simulink model "STEVE_ver28"  (R2022a)
settings: Solver=VariableStepAuto  StartTime=0.0  StopTime=Stop_Time  FixedStep=0.000001  RelTol=1e-5
values from neighbouring files (symbols this model uses):
  Bed_ave_OD = (1+Bed_ins_OD)/2    (= 1.667)    [STEVE_initialization.m]    (also in STEVE_running.m = (1+Bed_ins_OD)/2; STEVE_v4_C1Demo_2023_Nominal.m)
  Bed_ins_OD = 2.334    [STEVE_initialization.m]    (also in STEVE_v4_C1Demo_2023_Nominal.m)
  Bed_thickness = 0.049    [STEVE_initialization.m]    (also in STEVE_v4_C1Demo_2023_Nominal.m)
  Belimo_Cv = 16    [STEVE_initialization.m]    (also in STEVE_v4_C1Demo_2023_Nominal.m)
  flow_rate = 8    [STEVE_initialization.m]    (also in STEVE_v4_C1Demo_2023_Nominal.m)
  Heat_ads = 40000    [STEVE_initialization.m]    (also in STEVE_v4_C1Demo_2023_Nominal.m)
  Heater_output = 85.3    [STEVE_initialization.m]    (also in STEVE_v4_C1Demo_2023_Nominal.m)
  L = 0.508    [STEVE_initialization.m]    (also in STEVE_v4_C1Demo_2023_Nominal.m)
  L_inch = L*39.3701    (= 20.0000108)    [STEVE_initialization.m]    (also in STEVE_v4_C1Demo_2023_Nominal.m)
  max_temp = 200+273.15    (= 473.15)    [STEVE_initialization.m]    (also in STEVE_v4_C1Demo_2023_Nominal.m)
  mesh_size = 15    [STEVE_initialization.m]    (also in STEVE_v4_C1Demo_2023_Nominal.m)
  Pipe_ave_HD = (pipe_HD+0.5)/2    (= 0.465)    [STEVE_initialization.m]    (also in STEVE_running.m = (pipe_HD+0.5)/2; STEVE_v4_C1Demo_2023_Nominal.m)
  pipe_HD = 0.43    [STEVE_initialization.m]    (also in STEVE_v4_C1Demo_2023_Nominal.m)
  Ramp_rate = 0.0833    [STEVE_initialization.m]    (also in STEVE_v4_C1Demo_2023_Nominal.m)
  room_pressure = 13.3    [STEVE_initialization.m]    (also in STEVE_v4_C1Demo_2023_Nominal.m)
  t_Total = Adsorption_time + FlowStop_time + Valve_close_Time + Select_valve_close_Time + Pump_down_time + Desorption_time + SelectValve_open_Time + Valve_open_Time    (= 9635)    [STEVE_initialization.m]    (also in STEVE_running.m = Adsorption_time + FlowStop_time + Valve_close_Time + Select_; STEVE_v4_C1Demo_2023_Nominal.m)
libraries: fl_lib x229, nesl_utility x75, slpidlib x2
(part 3 of 5)

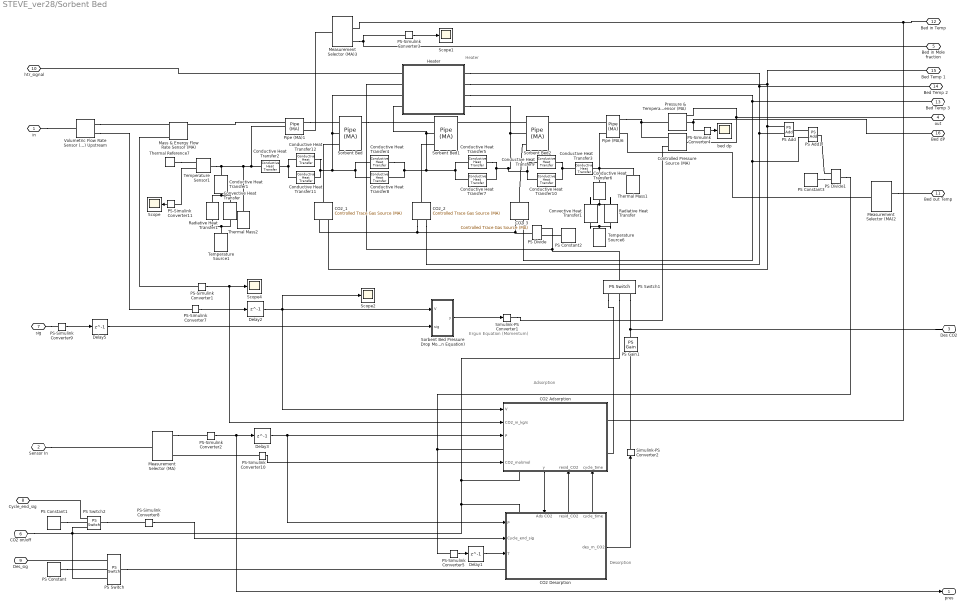
== system STEVE_ver28/Sorbent Bed ==
  note: Adsorption
  note: Desorption
  note: Heater
  note: Ergun Equation
      | (Momentum)
  CO2 Adsorption : Subsystem
      settings: PortSchema="{\"entries\":[{\"content\":{\"sides\":[{\"content\":{\"connectorIds\":[\"In1\",\"In2\",\"In3\",\"LConn1\",\"In4\"]},\"type\":\"ConnectorPlacement.EquallySpacedRectSide\",\"uuid\":\"fb5d8689-8c7c-41c6-b33a-026ebdfeda46\"},{\"content\":{\"connectorIds\":[\"RConn1\",\"RConn2\"],\"side\":\"RIGHT\"},\"type\":\"ConnectorPlacement.EquallySpacedRectSide\",\"uuid\":\"e615a398-5db1-42bf-ba80-688914a64f02\"},{\"content\":{\"connectorIds\":[],\"side\":\"TOP\"},\"type\":\"ConnectorPlacement.EquallySpacedRectSide\",\"uuid\":\"9c645526-20b8-4187-b1de-a01e982b301c\"},{\"content\":{\"connectorIds\":[\"RConn3\",\"Out1\",\"In5\",\"In6\"],\"side\":\"BOTTOM\"},\"type\":\"ConnectorPlacement.EquallySpacedRectSide\",\"uuid\":\"6466ec51-34c2-43b0-b46d-13f7eb07024c\"}]},\"type\":\"ConnectorPlacement.EquallySpacedConnector\",\"uuid\":\"b40ef80e-51c9-40d8-be75-3e6ecf2a6433\"}],\"packageUris\":[\"http://schema.mathworks.com/mf0/Connector/R2020b\"],\"version\":\"1.0\"}"
  CO2 Desorption : Subsystem
      settings: PortSchema="{\"entries\":[{\"content\":{\"sides\":[{\"content\":{\"connectorIds\":[\"In1\",\"In2\",\"In3\",\"LConn1\"]},\"type\":\"ConnectorPlacement.EquallySpacedRectSide\",\"uuid\":\"c0a19cc0-55b6-4f26-88f6-d4532b770ac9\"},{\"content\":{\"connectorIds\":[\"Out1\"],\"side\":\"RIGHT\"},\"type\":\"ConnectorPlacement.EquallySpacedRectSide\",\"uuid\":\"04c46a21-a116-4a66-b667-6b06cdc38df3\"},{\"content\":{\"connectorIds\":[\"LConn2\",\"In4\",\"Out2\",\"Out3\"],\"side\":\"TOP\"},\"type\":\"ConnectorPlacement.EquallySpacedRectSide\",\"uuid\":\"2474eb99-1ff9-473d-8974-056a2586b2d8\"}]},\"type\":\"ConnectorPlacement.EquallySpacedConnector\",\"uuid\":\"155b9182-f960-4b43-b6e5-30b3ea77ead6\"}],\"packageUris\":[\"http://schema.mathworks.com/mf0/Connector/R2020b\"],\"version\":\"1.0\"}"
  CO2_1 : fl_lib/Moist Air/Sources/Moisture & Trace Gas Sources/Controlled Trace Gas Source (MA)  Phi_S_specify=off  Phi_S_priority=None  Phi_S=0 kW  Phi_S_nominal_specify=off  Phi_S_nominal_unit=kW  Phi_S_nominal_value=1  mdot_g_S_specify=off  mdot_g_S_priority=None  mdot_g_S=0 kg/s  mdot_g_S_nominal_specify=off  mdot_g_S_nominal_unit=kg/s  mdot_g_S_nominal_value=1
      settings: SourceProductBaseCode=PW,SS,VE  InternalSimscapePortConfiguration="{\"Bottom\":[],\"Left\":[{\"id\":\"S\",\"label\":\"S\",\"type\":\"foundation.moist_air.moist_air_source\"}],\"Right\":[{\"id\":\"M\",\"label\":\"M\",\"type\":\"input\"},{\"id\":\"T\",\"label\":\"T\",\"type\":\"input\"}],\"Top\":[]}"
  CO2_2 : fl_lib/Moist Air/Sources/Moisture & Trace Gas Sources/Controlled Trace Gas Source (MA)  Phi_S_specify=off  Phi_S_priority=None  Phi_S=0 kW  Phi_S_nominal_specify=off  Phi_S_nominal_unit=kW  Phi_S_nominal_value=1  mdot_g_S_specify=off  mdot_g_S_priority=None  mdot_g_S=0 kg/s  mdot_g_S_nominal_specify=off  mdot_g_S_nominal_unit=kg/s  mdot_g_S_nominal_value=1
      settings: SourceProductBaseCode=PW,SS,VE  InternalSimscapePortConfiguration="{\"Bottom\":[],\"Left\":[{\"id\":\"S\",\"label\":\"S\",\"type\":\"foundation.moist_air.moist_air_source\"}],\"Right\":[{\"id\":\"M\",\"label\":\"M\",\"type\":\"input\"},{\"id\":\"T\",\"label\":\"T\",\"type\":\"input\"}],\"Top\":[]}"
  CO2_3 : fl_lib/Moist Air/Sources/Moisture & Trace Gas Sources/Controlled Trace Gas Source (MA)  Phi_S_specify=off  Phi_S_priority=None  Phi_S=0 kW  Phi_S_nominal_specify=off  Phi_S_nominal_unit=kW  Phi_S_nominal_value=1  mdot_g_S_specify=off  mdot_g_S_priority=None  mdot_g_S=0 kg/s  mdot_g_S_nominal_specify=off  mdot_g_S_nominal_unit=kg/s  mdot_g_S_nominal_value=1
      settings: SourceProductBaseCode=PW,SS,VE  InternalSimscapePortConfiguration="{\"Bottom\":[],\"Left\":[{\"id\":\"S\",\"label\":\"S\",\"type\":\"foundation.moist_air.moist_air_source\"}],\"Right\":[{\"id\":\"M\",\"label\":\"M\",\"type\":\"input\"},{\"id\":\"T\",\"label\":\"T\",\"type\":\"input\"}],\"Top\":[]}"
  Conductive Heat Transfer1 : fl_lib/Thermal/Thermal Elements/Conductive Heat Transfer  area=2*pi*(1.531/2)*1.2 in^2  thickness=(1.531-Bed_thickness*2-pipe_HD)/2 in  th_cond=pipe_tc W/(m*K)  T_specify=off  T_priority=None  T=0 K  T_nominal_specify=off  T_nominal_unit=K  T_nominal_value=1  Q_specify=off  Q_priority=None  Q=0 W  Q_nominal_specify=off  Q_nominal_unit=W  Q_nominal_value=1
      settings: SourceProductBaseCode=PW,SS,VE
  Conductive Heat Transfer10 : fl_lib/Thermal/Thermal Elements/Conductive Heat Transfer  area=pi*(0.902/2)^2 in^2  thickness=20/3 in  th_cond=0.15 W/(m*K)  T_specify=off  T_priority=None  T=0 K  T_nominal_specify=off  T_nominal_unit=K  T_nominal_value=1  Q_specify=off  Q_priority=None  Q=0 W  Q_nominal_specify=off  Q_nominal_unit=W  Q_nominal_value=1
      settings: SourceProductBaseCode=PW,SS,VE
  Conductive Heat Transfer11 : fl_lib/Thermal/Thermal Elements/Conductive Heat Transfer  area=pi*(0.902/2)^2 in^2  thickness=20/3 in  th_cond=0.15 W/(m*K)  T_specify=off  T_priority=None  T=0 K  T_nominal_specify=off  T_nominal_unit=K  T_nominal_value=1  Q_specify=off  Q_priority=None  Q=0 W  Q_nominal_specify=off  Q_nominal_unit=W  Q_nominal_value=1
      settings: SourceProductBaseCode=PW,SS,VE
  Conductive Heat Transfer12 : fl_lib/Thermal/Thermal Elements/Conductive Heat Transfer  area=2*pi*(0.902/2)*Bed_thickness in^2  thickness=20/3 in  th_cond=pipe_tc W/(m*K)  T_specify=off  T_priority=None  T=0 K  T_nominal_specify=off  T_nominal_unit=K  T_nominal_value=1  Q_specify=off  Q_priority=None  Q=0 W  Q_nominal_specify=off  Q_nominal_unit=W  Q_nominal_value=1
      settings: SourceProductBaseCode=PW,SS,VE
  Conductive Heat Transfer2 : fl_lib/Thermal/Thermal Elements/Conductive Heat Transfer  area=2*pi*(0.902/2)*Bed_thickness in^2  thickness=1.2 in  th_cond=pipe_tc W/(m*K)  T_specify=off  T_priority=None  T=0 K  T_nominal_specify=off  T_nominal_unit=K  T_nominal_value=1  Q_specify=off  Q_priority=None  Q=0 W  Q_nominal_specify=off  Q_nominal_unit=W  Q_nominal_value=1
      settings: SourceProductBaseCode=PW,SS,VE
  Conductive Heat Transfer3 : fl_lib/Thermal/Thermal Elements/Conductive Heat Transfer  area=2*pi*(0.902/2)*Bed_thickness in^2  thickness=1.2 in  th_cond=pipe_tc W/(m*K)  T_specify=off  T_priority=None  T=0 K  T_nominal_specify=off  T_nominal_unit=K  T_nominal_value=1  Q_specify=off  Q_priority=None  Q=0 W  Q_nominal_specify=off  Q_nominal_unit=W  Q_nominal_value=1
      settings: SourceProductBaseCode=PW,SS,VE
  Conductive Heat Transfer4 : fl_lib/Thermal/Thermal Elements/Conductive Heat Transfer  area=2*pi*(0.902/2)*Bed_thickness in^2  thickness=20/(3*2) in  th_cond=pipe_tc W/(m*K)  T_specify=off  T_priority=None  T=0 K  T_nominal_specify=off  T_nominal_unit=K  T_nominal_value=1  Q_specify=off  Q_priority=None  Q=0 W  Q_nominal_specify=off  Q_nominal_unit=W  Q_nominal_value=1
      settings: SourceProductBaseCode=PW,SS,VE
  Conductive Heat Transfer5 : fl_lib/Thermal/Thermal Elements/Conductive Heat Transfer  area=2*pi*(0.902/2)*Bed_thickness in^2  thickness=20/(3*2) in  th_cond=pipe_tc W/(m*K)  T_specify=off  T_priority=None  T=0 K  T_nominal_specify=off  T_nominal_unit=K  T_nominal_value=1  Q_specify=off  Q_priority=None  Q=0 W  Q_nominal_specify=off  Q_nominal_unit=W  Q_nominal_value=1
      settings: SourceProductBaseCode=PW,SS,VE
  Conductive Heat Transfer6 : fl_lib/Thermal/Thermal Elements/Conductive Heat Transfer  area=2*pi*(1.531/2)*1.2 in^2  thickness=(1.531-Bed_thickness*2-pipe_HD)/2 in  th_cond=pipe_tc W/(m*K)  T_specify=off  T_priority=None  T=0 K  T_nominal_specify=off  T_nominal_unit=K  T_nominal_value=1  Q_specify=off  Q_priority=None  Q=0 W  Q_nominal_specify=off  Q_nominal_unit=W  Q_nominal_value=1
      settings: SourceProductBaseCode=PW,SS,VE
  Conductive Heat Transfer7 : fl_lib/Thermal/Thermal Elements/Conductive Heat Transfer  area=pi*(0.902/2)^2 in^2  thickness=20/(3*2) in  th_cond=0.15 W/(m*K)  T_specify=off  T_priority=None  T=0 K  T_nominal_specify=off  T_nominal_unit=K  T_nominal_value=1  Q_specify=off  Q_priority=None  Q=0 W  Q_nominal_specify=off  Q_nominal_unit=W  Q_nominal_value=1
      settings: SourceProductBaseCode=PW,SS,VE
  Conductive Heat Transfer8 : fl_lib/Thermal/Thermal Elements/Conductive Heat Transfer  area=pi*(0.902/2)^2 in^2  thickness=20/(3*2) in  th_cond=0.15 W/(m*K)  T_specify=off  T_priority=None  T=0 K  T_nominal_specify=off  T_nominal_unit=K  T_nominal_value=1  Q_specify=off  Q_priority=None  Q=0 W  Q_nominal_specify=off  Q_nominal_unit=W  Q_nominal_value=1
      settings: SourceProductBaseCode=PW,SS,VE
  Conductive Heat Transfer9 : fl_lib/Thermal/Thermal Elements/Conductive Heat Transfer  area=2*pi*(0.902/2)*Bed_thickness in^2  thickness=20/3 in  th_cond=pipe_tc W/(m*K)  T_specify=off  T_priority=None  T=0 K  T_nominal_specify=off  T_nominal_unit=K  T_nominal_value=1  Q_specify=off  Q_priority=None  Q=0 W  Q_nominal_specify=off  Q_nominal_unit=W  Q_nominal_value=1
      settings: SourceProductBaseCode=PW,SS,VE
  Controlled Pressure Source (MA) : fl_lib/Moist Air/Sources/Controlled Pressure Source (MA)  power_spec=foundation.enum.power_spec.none  area_A=0.639 in^2  area_B=0.639 in^2
      settings: SourceProductBaseCode=PW,SS,VE  InternalSimscapePortConfiguration="{\"Bottom\":[],\"Left\":[{\"id\":\"A\",\"label\":\"A\",\"type\":\"foundation.moist_air.moist_air\"},{\"id\":\"P\",\"label\":\"P\",\"type\":\"input\"}],\"Right\":[{\"id\":\"B\",\"label\":\"B\",\"type\":\"foundation.moist_air.moist_air\"}],\"Top\":[]}"
  Convective Heat Transfer : fl_lib/Thermal/Thermal Elements/Convective Heat Transfer  area=2*pi*(1.531/2)*1.2 in^2  heat_tr_coeff=5 W/(K*m^2)  T_specify=off  T_priority=None  T=0 K  T_nominal_specify=off  T_nominal_unit=K  T_nominal_value=1  Q_specify=off  Q_priority=None  Q=0 W  Q_nominal_specify=off  Q_nominal_unit=W  Q_nominal_value=1
      settings: SourceProductBaseCode=PW,SS,VE
  Convective Heat Transfer1 : fl_lib/Thermal/Thermal Elements/Convective Heat Transfer  area=2*pi*(1.531/2)*1.2 in^2  heat_tr_coeff=5 W/(K*m^2)  T_specify=off  T_priority=None  T=0 K  T_nominal_specify=off  T_nominal_unit=K  T_nominal_value=1  Q_specify=off  Q_priority=None  Q=0 W  Q_nominal_specify=off  Q_nominal_unit=W  Q_nominal_value=1
      settings: SourceProductBaseCode=PW,SS,VE
  Delay1 : Delay  DelayLength=1  InitialCondition=293.15
  Delay2 : Delay  DelayLength=1  InitialCondition=0.00013
  Delay3 : Delay  DelayLength=1  InitialCondition=91700
  Delay5 : Delay  DelayLength=1  InitialCondition=0
  Heater : Subsystem
  Mass & Energy Flow Rate Sensor (MA) : fl_lib/Moist Air/Sensors/Mass & Energy Flow Rate Sensor (MA)
      settings: SourceProductBaseCode=PW,SS,VE  InternalSimscapePortConfiguration="{\"Bottom\":[],\"Left\":[{\"id\":\"A\",\"label\":\"A\",\"type\":\"foundation.moist_air.moist_air\"},{\"id\":\"Mw\",\"label\":\"Mw\",\"type\":\"output\"},{\"id\":\"Mg\",\"label\":\"Mg\",\"type\":\"output\"}],\"Right\":[{\"id\":\"B\",\"label\":\"B\",\"type\":\"foundation.moist_air.moist_air\"},{\"id\":\"M\",\"label\":\"M\",\"type\":\"output\"},{\"id\":\"PHI\",\"label\":\"Phi\",\"type\":\"output\"}],\"Top\":[]}"
  Measurement Selector (MA) : fl_lib/Moist Air/Sensors/Measurement Selector (MA)  moisture_spec=foundation.enum.moisture_spec.relative_humidity  trace_gas_spec=foundation.enum.trace_gas_spec.mole_fraction
      settings: SourceProductBaseCode=PW,SS,VE
  Measurement Selector (MA)2 : fl_lib/Moist Air/Sensors/Measurement Selector (MA)  moisture_spec=foundation.enum.moisture_spec.relative_humidity  trace_gas_spec=foundation.enum.trace_gas_spec.mole_fraction
      settings: SourceProductBaseCode=PW,SS,VE
  Measurement Selector (MA)3 : fl_lib/Moist Air/Sensors/Measurement Selector (MA)  moisture_spec=foundation.enum.moisture_spec.relative_humidity  trace_gas_spec=foundation.enum.trace_gas_spec.mole_fraction
      settings: SourceProductBaseCode=PW,SS,VE
  PS Add : fl_lib/Physical Signals/Functions/PS Add
      settings: SourceProductBaseCode=PW,SS,VE
  PS Add1 : fl_lib/Physical Signals/Functions/PS Add
      settings: SourceProductBaseCode=PW,SS,VE
  PS Constant : fl_lib/Physical Signals/Sources/PS Constant  constant=1
      settings: SourceProductBaseCode=PW,SS,VE
  PS Constant1 : fl_lib/Physical Signals/Sources/PS Constant  constant=1
      settings: SourceProductBaseCode=PW,SS,VE
  PS Constant2 : fl_lib/Physical Signals/Sources/PS Constant  constant=3
      settings: SourceProductBaseCode=PW,SS,VE
  PS Constant3 : fl_lib/Physical Signals/Sources/PS Constant  constant=3
      settings: SourceProductBaseCode=PW,SS,VE
  PS Divide : fl_lib/Physical Signals/Functions/PS Divide
      settings: SourceProductBaseCode=PW,SS,VE
  PS Divide1 : fl_lib/Physical Signals/Functions/PS Divide
      settings: SourceProductBaseCode=PW,SS,VE
  PS Gain1 : fl_lib/Physical Signals/Functions/PS Gain  gain=1
      settings: SourceProductBaseCode=PW,SS,VE
  PS Switch : fl_lib/Physical Signals/Nonlinear Operators/PS Switch  Threshold=1
      settings: SourceProductBaseCode=PW,SS,VE  InternalSimscapePortConfiguration="{\"Bottom\":[],\"Left\":[{\"id\":\"I1\",\"label\":\"\",\"type\":\"input\"},{\"id\":\"I2\",\"label\":\"\",\"type\":\"input\"},{\"id\":\"I3\",\"label\":\"\",\"type\":\"input\"}],\"Right\":[{\"id\":\"O\",\"label\":\"\",\"type\":\"output\"}],\"Top\":[]}"
  PS Switch1 : fl_lib/Physical Signals/Nonlinear Operators/PS Switch  Threshold=1
      settings: SourceProductBaseCode=PW,SS,VE  InternalSimscapePortConfiguration="{\"Bottom\":[],\"Left\":[{\"id\":\"I1\",\"label\":\"\",\"type\":\"input\"},{\"id\":\"I2\",\"label\":\"\",\"type\":\"input\"},{\"id\":\"I3\",\"label\":\"\",\"type\":\"input\"}],\"Right\":[{\"id\":\"O\",\"label\":\"\",\"type\":\"output\"}],\"Top\":[]}"
  PS Switch2 : fl_lib/Physical Signals/Nonlinear Operators/PS Switch  Threshold=1
      settings: SourceProductBaseCode=PW,SS,VE  InternalSimscapePortConfiguration="{\"Bottom\":[],\"Left\":[{\"id\":\"I1\",\"label\":\"\",\"type\":\"input\"},{\"id\":\"I2\",\"label\":\"\",\"type\":\"input\"},{\"id\":\"I3\",\"label\":\"\",\"type\":\"input\"}],\"Right\":[{\"id\":\"O\",\"label\":\"\",\"type\":\"output\"}],\"Top\":[]}"
  PS-Simulink Converter{1..3,5,7..11} (9 alike) : nesl_utility/PS-Simulink Converter  PhysicalDomain=network_engine_domain  SubClassName=ps_output  LeftPortType=input  RightPortType=output  PseudoPeriodic=off  Frequencies=[]  VectorFormat=1-D array  Unit=inherit  AffineConversion=off
      settings: SourceProductBaseCode=SS,PW,VE
  PS-Simulink Converter4 : nesl_utility/PS-Simulink Converter  PhysicalDomain=network_engine_domain  SubClassName=ps_output  LeftPortType=input  RightPortType=output  PseudoPeriodic=off  Frequencies=[]  VectorFormat=1-D array  Unit=Pa  AffineConversion=off
      settings: SourceProductBaseCode=SS,PW,VE
  Pipe (MA)1 : fl_lib/Moist Air/Elements/Pipe (MA)  length=1.2 in  area=pi*(0.902/2)^2 in^2  Dh=0.902 in  length_add=0.1 m  roughness=roughness m  Re_lam=2000  Re_tur=4000  shape_factor=64  Nu_lam=3.66  RH_ws=1  time_constant=1e-3 s  moisture_trace_gas_source=foundation.enum.moisture_trace_gas_source.controlled  moisture_source_spec=foundation.enum.moisture_source_spec.vapor  moisture_mass_flow=0 kg/s  moisture_temperature_spec=foundation.enum.temperature_spec.atmospheric  moisture_temperature=293.15 K  trace_gas_mass_flow=0 kg/s  trace_gas_temperature_spec=foundation.enum.temperature_spec.atmospheric  trace_gas_temperature=293.15 K  p_I_specify=off  p_I_priority=High  p_I=0.101325 MPa  p_I_nominal_specify=off  p_I_nominal_unit=MPa  p_I_nominal_value=1  T_I_specify=off  T_I_priority=High  T_I=293.15 K  T_I_nominal_specify=off  T_I_nominal_unit=K  T_I_nominal_value=1  RH_I_specify=off  RH_I_priority=High  RH_I=0  RH_I_nominal_specify=off  RH_I_nominal_unit=1  RH_I_nominal_value=1  x_w_I_specify=off  x_w_I_priority=None  x_w_I=0  x_w_I_nominal_specify=off  x_w_I_nominal_unit=1  x_w_I_nominal_value=1  y_w_I_specify=off  y_w_I_priority=None  y_w_I=0  y_w_I_nominal_specify=off  y_w_I_nominal_unit=1  y_w_I_nominal_value=1  HR_I_specify=off  HR_I_priority=None  HR_I=0  HR_I_nominal_specify=off  HR_I_nominal_unit=1  HR_I_nominal_value=1  x_g_I_specify=off  x_g_I_priority=High  x_g_I=0  x_g_I_nominal_specify=off  x_g_I_nominal_unit=1  x_g_I_nominal_value=1  y_g_I_specify=off  y_g_I_priority=None  y_g_I=0  y_g_I_nominal_specify=off  y_g_I_nominal_unit=1  y_g_I_nominal_value=1
      settings: SourceProductBaseCode=PW,SS,VE  InternalSimscapePortConfiguration="{\"Bottom\":[],\"Left\":[{\"id\":\"A\",\"label\":\"A\",\"type\":\"foundation.moist_air.moist_air\"},{\"id\":\"H\",\"label\":\"H\",\"type\":\"foundation.thermal.thermal\"},{\"id\":\"S\",\"label\":\"S\",\"type\":\"foundation.moist_air.moist_air_source\"}],\"Right\":[{\"id\":\"B\",\"label\":\"B\",\"type\":\"foundation.moist_air.moist_air\"},{\"id\":\"W\",\"label\":\"W\",\"type\":\"output\"},{\"id\":\"F\",\"label\":\"F\",\"type\":\"output\"}],\"Top\":[]}"
  Pipe (MA)6 : fl_lib/Moist Air/Elements/Pipe (MA)  length=1.2 in  area=pi*(0.902/2)^2 in^2  Dh=0.902 in  length_add=0.1 m  roughness=roughness m  Re_lam=2000  Re_tur=4000  shape_factor=64  Nu_lam=3.66  RH_ws=1  time_constant=1e-3 s  moisture_trace_gas_source=foundation.enum.moisture_trace_gas_source.none  moisture_source_spec=foundation.enum.moisture_source_spec.vapor  moisture_mass_flow=0 kg/s  moisture_temperature_spec=foundation.enum.temperature_spec.atmospheric  moisture_temperature=293.15 K  trace_gas_mass_flow=0 kg/s  trace_gas_temperature_spec=foundation.enum.temperature_spec.atmospheric  trace_gas_temperature=293.15 K  p_I_specify=off  p_I_priority=High  p_I=0.101325 MPa  p_I_nominal_specify=off  p_I_nominal_unit=MPa  p_I_nominal_value=1  T_I_specify=off  T_I_priority=High  T_I=293.15 K  T_I_nominal_specify=off  T_I_nominal_unit=K  T_I_nominal_value=1  RH_I_specify=off  RH_I_priority=High  RH_I=0  RH_I_nominal_specify=off  RH_I_nominal_unit=1  RH_I_nominal_value=1  x_w_I_specify=off  x_w_I_priority=None  x_w_I=0  x_w_I_nominal_specify=off  x_w_I_nominal_unit=1  x_w_I_nominal_value=1  y_w_I_specify=off  y_w_I_priority=None  y_w_I=0  y_w_I_nominal_specify=off  y_w_I_nominal_unit=1  y_w_I_nominal_value=1  HR_I_specify=off  HR_I_priority=None  HR_I=0  HR_I_nominal_specify=off  HR_I_nominal_unit=1  HR_I_nominal_value=1  x_g_I_specify=off  x_g_I_priority=High  x_g_I=0  x_g_I_nominal_specify=off  x_g_I_nominal_unit=1  x_g_I_nominal_value=1  y_g_I_specify=off  y_g_I_priority=None  y_g_I=0  y_g_I_nominal_specify=off  y_g_I_nominal_unit=1  y_g_I_nominal_value=1
      settings: SourceProductBaseCode=PW,SS,VE
  Pressure & Temperature Sensor (MA) : fl_lib/Moist Air/Sensors/Pressure & Temperature Sensor (MA)
      settings: SourceProductBaseCode=PW,SS,VE  InternalSimscapePortConfiguration="{\"Bottom\":[],\"Left\":[{\"id\":\"A\",\"label\":\"A\",\"type\":\"foundation.moist_air.moist_air\"}],\"Right\":[{\"id\":\"B\",\"label\":\"B\",\"type\":\"foundation.moist_air.moist_air\"},{\"id\":\"P\",\"label\":\"P\",\"type\":\"output\"},{\"id\":\"T\",\"label\":\"T\",\"type\":\"output\"}],\"Top\":[]}"
  Radiative Heat Transfer : fl_lib/Thermal/Thermal Elements/Radiative Heat Transfer  area=2*pi*(1.531/2)*1.2 in^2  rad_tr_coeff=3.97e-9 W/(K^4*m^2)  T_specify=off  T_priority=None  T=0 K  T_nominal_specify=off  T_nominal_unit=K  T_nominal_value=1  Q_specify=off  Q_priority=None  Q=0 W  Q_nominal_specify=off  Q_nominal_unit=W  Q_nominal_value=1
      settings: SourceProductBaseCode=PW,SS,VE  InternalSimscapePortConfiguration="{\"Bottom\":[],\"Left\":[{\"id\":\"A\",\"label\":\"A\",\"type\":\"foundation.thermal.thermal\"}],\"Right\":[{\"id\":\"B\",\"label\":\"B\",\"type\":\"foundation.thermal.thermal\"}],\"Top\":[]}"
  Radiative Heat Transfer1 : fl_lib/Thermal/Thermal Elements/Radiative Heat Transfer  area=2*pi*(1.531/2)*1.2 in^2  rad_tr_coeff=3.97e-9 W/(K^4*m^2)  T_specify=off  T_priority=None  T=0 K  T_nominal_specify=off  T_nominal_unit=K  T_nominal_value=1  Q_specify=off  Q_priority=None  Q=0 W  Q_nominal_specify=off  Q_nominal_unit=W  Q_nominal_value=1
      settings: SourceProductBaseCode=PW,SS,VE  InternalSimscapePortConfiguration="{\"Bottom\":[],\"Left\":[{\"id\":\"A\",\"label\":\"A\",\"type\":\"foundation.thermal.thermal\"}],\"Right\":[{\"id\":\"B\",\"label\":\"B\",\"type\":\"foundation.thermal.thermal\"}],\"Top\":[]}"
  Scope{,1..2,4} (4 alike) : Scope
  Simulink-PS Converter1 : nesl_utility/Simulink-PS Converter  PhysicalDomain=network_engine_domain  SubClassName=ps_input  LeftPortType=input  RightPortType=output  PseudoPeriodic=off  Frequencies=[]  NoiseDistribution=none  NoiseParameters=[]  Unit=Pa  AffineConversion=off  FilteringAndDerivatives=provide  SimscapeFilterOrder=1  InputFilterTimeConstant=0.001  UdotUserProvided=0
      settings: SourceProductBaseCode=SS,PW,VE
  Simulink-PS Converter2 : nesl_utility/Simulink-PS Converter  PhysicalDomain=network_engine_domain  SubClassName=ps_input  LeftPortType=input  RightPortType=output  PseudoPeriodic=off  Frequencies=[]  NoiseDistribution=none  NoiseParameters=[]  Unit=kg/s  AffineConversion=off  FilteringAndDerivatives=provide  SimscapeFilterOrder=1  InputFilterTimeConstant=0.001  UdotUserProvided=0
      settings: SourceProductBaseCode=SS,PW,VE
  Sorbent Bed : fl_lib/Moist Air/Elements/Pipe (MA)  length=L_inch/3 in  area=pi*(0.902/2)^2 in^2  Dh=0.902 in  length_add=0.1 m  roughness=roughness m  Re_lam=2000  Re_tur=4000  shape_factor=64  Nu_lam=3.66  RH_ws=1  time_constant=1e-3 s  moisture_trace_gas_source=foundation.enum.moisture_trace_gas_source.controlled  moisture_source_spec=foundation.enum.moisture_source_spec.vapor  moisture_mass_flow=0 kg/s  moisture_temperature_spec=foundation.enum.temperature_spec.atmospheric  moisture_temperature=293.15 K  trace_gas_mass_flow=0 kg/s  trace_gas_temperature_spec=foundation.enum.temperature_spec.atmospheric  trace_gas_temperature=293.15 K  p_I_specify=off  p_I_priority=High  p_I=0.101325 MPa  p_I_nominal_specify=off  p_I_nominal_unit=MPa  p_I_nominal_value=1  T_I_specify=off  T_I_priority=High  T_I=293.15 K  T_I_nominal_specify=off  T_I_nominal_unit=K  T_I_nominal_value=1  RH_I_specify=off  RH_I_priority=High  RH_I=0  RH_I_nominal_specify=off  RH_I_nominal_unit=1  RH_I_nominal_value=1  x_w_I_specify=off  x_w_I_priority=None  x_w_I=0  x_w_I_nominal_specify=off  x_w_I_nominal_unit=1  x_w_I_nominal_value=1  y_w_I_specify=off  y_w_I_priority=None  y_w_I=0  y_w_I_nominal_specify=off  y_w_I_nominal_unit=1  y_w_I_nominal_value=1  HR_I_specify=off  HR_I_priority=None  HR_I=0  HR_I_nominal_specify=off  HR_I_nominal_unit=1  HR_I_nominal_value=1  x_g_I_specify=off  x_g_I_priority=High  x_g_I=0  x_g_I_nominal_specify=off  x_g_I_nominal_unit=1  x_g_I_nominal_value=1  y_g_I_specify=off  y_g_I_priority=None  y_g_I=0  y_g_I_nominal_specify=off  y_g_I_nominal_unit=1  y_g_I_nominal_value=1
      settings: SourceProductBaseCode=PW,SS,VE  InternalSimscapePortConfiguration="{\"Bottom\":[],\"Left\":[{\"id\":\"A\",\"label\":\"A\",\"type\":\"foundation.moist_air.moist_air\"},{\"id\":\"H\",\"label\":\"H\",\"type\":\"foundation.thermal.thermal\"},{\"id\":\"S\",\"label\":\"S\",\"type\":\"foundation.moist_air.moist_air_source\"}],\"Right\":[{\"id\":\"B\",\"label\":\"B\",\"type\":\"foundation.moist_air.moist_air\"},{\"id\":\"W\",\"label\":\"W\",\"type\":\"output\"},{\"id\":\"F\",\"label\":\"F\",\"type\":\"output\"}],\"Top\":[]}"
  Sorbent Bed Pressure Drop Model (Ergun Equation) : MATLAB Function  TreatAsAtomicUnit=on
  Sorbent Bed1 : fl_lib/Moist Air/Elements/Pipe (MA)  length=L_inch/3 in  area=pi*(0.902/2)^2 in^2  Dh=0.902 in  length_add=0.1 m  roughness=roughness m  Re_lam=2000  Re_tur=4000  shape_factor=64  Nu_lam=3.66  RH_ws=1  time_constant=1e-3 s  moisture_trace_gas_source=foundation.enum.moisture_trace_gas_source.controlled  moisture_source_spec=foundation.enum.moisture_source_spec.vapor  moisture_mass_flow=0 kg/s  moisture_temperature_spec=foundation.enum.temperature_spec.atmospheric  moisture_temperature=293.15 K  trace_gas_mass_flow=0 kg/s  trace_gas_temperature_spec=foundation.enum.temperature_spec.atmospheric  trace_gas_temperature=293.15 K  p_I_specify=off  p_I_priority=High  p_I=0.101325 MPa  p_I_nominal_specify=off  p_I_nominal_unit=MPa  p_I_nominal_value=1  T_I_specify=off  T_I_priority=High  T_I=293.15 K  T_I_nominal_specify=off  T_I_nominal_unit=K  T_I_nominal_value=1  RH_I_specify=off  RH_I_priority=High  RH_I=0  RH_I_nominal_specify=off  RH_I_nominal_unit=1  RH_I_nominal_value=1  x_w_I_specify=off  x_w_I_priority=None  x_w_I=0  x_w_I_nominal_specify=off  x_w_I_nominal_unit=1  x_w_I_nominal_value=1  y_w_I_specify=off  y_w_I_priority=None  y_w_I=0  y_w_I_nominal_specify=off  y_w_I_nominal_unit=1  y_w_I_nominal_value=1  HR_I_specify=off  HR_I_priority=None  HR_I=0  HR_I_nominal_specify=off  HR_I_nominal_unit=1  HR_I_nominal_value=1  x_g_I_specify=off  x_g_I_priority=High  x_g_I=0  x_g_I_nominal_specify=off  x_g_I_nominal_unit=1  x_g_I_nominal_value=1  y_g_I_specify=off  y_g_I_priority=None  y_g_I=0  y_g_I_nominal_specify=off  y_g_I_nominal_unit=1  y_g_I_nominal_value=1
      settings: SourceProductBaseCode=PW,SS,VE  InternalSimscapePortConfiguration="{\"Bottom\":[],\"Left\":[{\"id\":\"A\",\"label\":\"A\",\"type\":\"foundation.moist_air.moist_air\"},{\"id\":\"H\",\"label\":\"H\",\"type\":\"foundation.thermal.thermal\"},{\"id\":\"S\",\"label\":\"S\",\"type\":\"foundation.moist_air.moist_air_source\"}],\"Right\":[{\"id\":\"B\",\"label\":\"B\",\"type\":\"foundation.moist_air.moist_air\"},{\"id\":\"W\",\"label\":\"W\",\"type\":\"output\"},{\"id\":\"F\",\"label\":\"F\",\"type\":\"output\"}],\"Top\":[]}"
  Sorbent Bed2 : fl_lib/Moist Air/Elements/Pipe (MA)  length=L_inch/3 in  area=pi*(0.902/2)^2 in^2  Dh=0.902 in  length_add=0.1 m  roughness=roughness m  Re_lam=2000  Re_tur=4000  shape_factor=64  Nu_lam=3.66  RH_ws=1  time_constant=1e-3 s  moisture_trace_gas_source=foundation.enum.moisture_trace_gas_source.controlled  moisture_source_spec=foundation.enum.moisture_source_spec.vapor  moisture_mass_flow=0 kg/s  moisture_temperature_spec=foundation.enum.temperature_spec.atmospheric  moisture_temperature=293.15 K  trace_gas_mass_flow=0 kg/s  trace_gas_temperature_spec=foundation.enum.temperature_spec.atmospheric  trace_gas_temperature=293.15 K  p_I_specify=off  p_I_priority=High  p_I=0.101325 MPa  p_I_nominal_specify=off  p_I_nominal_unit=MPa  p_I_nominal_value=1  T_I_specify=off  T_I_priority=High  T_I=293.15 K  T_I_nominal_specify=off  T_I_nominal_unit=K  T_I_nominal_value=1  RH_I_specify=off  RH_I_priority=High  RH_I=0  RH_I_nominal_specify=off  RH_I_nominal_unit=1  RH_I_nominal_value=1  x_w_I_specify=off  x_w_I_priority=None  x_w_I=0  x_w_I_nominal_specify=off  x_w_I_nominal_unit=1  x_w_I_nominal_value=1  y_w_I_specify=off  y_w_I_priority=None  y_w_I=0  y_w_I_nominal_specify=off  y_w_I_nominal_unit=1  y_w_I_nominal_value=1  HR_I_specify=off  HR_I_priority=None  HR_I=0  HR_I_nominal_specify=off  HR_I_nominal_unit=1  HR_I_nominal_value=1  x_g_I_specify=off  x_g_I_priority=High  x_g_I=0  x_g_I_nominal_specify=off  x_g_I_nominal_unit=1  x_g_I_nominal_value=1  y_g_I_specify=off  y_g_I_priority=None  y_g_I=0  y_g_I_nominal_specify=off  y_g_I_nominal_unit=1  y_g_I_nominal_value=1
      settings: SourceProductBaseCode=PW,SS,VE  InternalSimscapePortConfiguration="{\"Bottom\":[],\"Left\":[{\"id\":\"A\",\"label\":\"A\",\"type\":\"foundation.moist_air.moist_air\"},{\"id\":\"H\",\"label\":\"H\",\"type\":\"foundation.thermal.thermal\"},{\"id\":\"S\",\"label\":\"S\",\"type\":\"foundation.moist_air.moist_air_source\"}],\"Right\":[{\"id\":\"B\",\"label\":\"B\",\"type\":\"foundation.moist_air.moist_air\"},{\"id\":\"W\",\"label\":\"W\",\"type\":\"output\"},{\"id\":\"F\",\"label\":\"F\",\"type\":\"output\"}],\"Top\":[]}"
  Temperature Sensor1 : fl_lib/Thermal/Thermal Sensors/Temperature Sensor
      settings: SourceProductBaseCode=PW,SS,VE
  Temperature Source1 : fl_lib/Thermal/Thermal Sources/Temperature Source  temperature=room_temp K
      settings: SourceProductBaseCode=PW,SS,VE
  Temperature Source6 : fl_lib/Thermal/Thermal Sources/Temperature Source  temperature=room_temp K
      settings: SourceProductBaseCode=PW,SS,VE
  Thermal Mass1 : fl_lib/Thermal/Thermal Elements/Thermal Mass  mass=216 g  sp_heat=490 J/kg/K  T_specify=off  T_priority=High  T=300 K  T_nominal_specify=off  T_nominal_unit=K  T_nominal_value=1  Q_specify=off  Q_priority=None  Q=0 W  Q_nominal_specify=off  Q_nominal_unit=W  Q_nominal_value=1
      settings: SourceProductBaseCode=PW,SS,VE
  Thermal Mass2 : fl_lib/Thermal/Thermal Elements/Thermal Mass  mass=216 g  sp_heat=490 J/kg/K  T_specify=off  T_priority=High  T=300 K  T_nominal_specify=off  T_nominal_unit=K  T_nominal_value=1  Q_specify=off  Q_priority=None  Q=0 W  Q_nominal_specify=off  Q_nominal_unit=W  Q_nominal_value=1
      settings: SourceProductBaseCode=PW,SS,VE
  Thermal Reference7 : fl_lib/Thermal/Thermal Elements/Thermal Reference
      settings: SourceProductBaseCode=PW,SS,VE
  Volumetric Flow Rate Sensor (MA) Upstream : fl_lib/Moist Air/Sensors/Volumetric Flow Rate Sensor (MA)  volumetric_flow_conditions=foundation.enum.volumetric_flow_conditions.actual  p_std=0.101325 MPa  T_std=20 degC  RH_std=0.65
      settings: SourceProductBaseCode=PW,SS,VE  InternalSimscapePortConfiguration="{\"Bottom\":[],\"Left\":[{\"id\":\"A\",\"label\":\"A\",\"type\":\"foundation.moist_air.moist_air\"}],\"Right\":[{\"id\":\"B\",\"label\":\"B\",\"type\":\"foundation.moist_air.moist_air\"},{\"id\":\"V\",\"label\":\"V\",\"type\":\"output\"}],\"Top\":[]}"
  bed dp : Scope
  in : PMIOPort  Side=Left
  Sensor In : PMIOPort  Port=2  Side=Left
  Des CO2 : PMIOPort  Port=3  Side=Left
  out : PMIOPort  Port=4  Side=Right
  Bed in Mole fraction : PMIOPort  Port=5  Side=Right
  CO2 on/off : PMIOPort  Port=6  Side=Right
  sig : PMIOPort  Port=7  Side=Right
  Cycle_end_sig : PMIOPort  Port=8  Side=Right
  Des_sig : PMIOPort  Port=9  Side=Right
  htr_signal : PMIOPort  Port=10  Side=Right
  Bed out Temp : PMIOPort  Port=11  Side=Right
  "Bed in Temp " : PMIOPort  Port=12  Side=Right
  Bed Temp 3 : PMIOPort  Port=13  Side=Right
  Bed Temp 2 : PMIOPort  Port=14  Side=Right
  Bed Temp 1 : PMIOPort  Port=15  Side=Right
  Bed dP : PMIOPort  Port=16  Side=Right
  pres : Outport
  wires:
  Sorbent Bed Pressure Drop Model (Ergun Equation)/1(y) -> Simulink-PS Converter1/1
  PS-Simulink Converter1/1 -> Scope4/1, CO2 Adsorption/2(CO2_in_kg/s)
  Delay2/1 -> CO2 Adsorption/1(V), Sorbent Bed Pressure Drop Model (Ergun Equation)/1(V), Scope2/1
  PS-Simulink Converter7/1 -> Delay2/1
  PS-Simulink Converter3/1 -> Scope1/1
  Delay3/1 -> CO2 Adsorption/3(P), CO2 Desorption/1(P)
  PS-Simulink Converter2/1 -> Delay3/1, pres/1
  PS-Simulink Converter4/1 -> bed dp/1
  Delay1/1 -> CO2 Desorption/3(T)
  PS-Simulink Converter5/1 -> Delay1/1
  CO2 Desorption/1(des_m_CO2) -> Simulink-PS Converter2/1
  CO2 Adsorption/1(y) -> CO2 Desorption/4(Ads CO2)
  PS-Simulink Converter9/1 -> Delay5/1
  Delay5/1 -> Sorbent Bed Pressure Drop Model (Ergun Equation)/2(sig)
  PS-Simulink Converter10/1 -> CO2 Adsorption/4(CO2_mol/mol)
  PS-Simulink Converter8/1 -> CO2 Desorption/2(Cycle_end_sig)
  CO2 Desorption/2(resid_CO2) -> CO2 Adsorption/5(resid_CO2)
  PS-Simulink Converter11/1 -> Scope/1
  CO2 Desorption/3(cycle_time) -> CO2 Adsorption/6(cycle_time)
  connections:
  Pressure & Temperature Sensor (MA)/RConn1 -- out/RConn1 -- Controlled Pressure Source (MA)/RConn1
  Pressure & Temperature Sensor (MA)/RConn2 -- Bed dP/RConn1 -- PS-Simulink Converter4/LConn1
  Measurement Selector (MA)/RConn1 -- PS-Simulink Converter2/LConn1
  Sensor In/RConn1 -- Measurement Selector (MA)/LConn1
  Volumetric Flow Rate Sensor (MA) Upstream/RConn1 -- Mass & Energy Flow Rate Sensor (MA)/LConn1
  in/RConn1 -- Volumetric Flow Rate Sensor (MA) Upstream/LConn1
  Simulink-PS Converter1/RConn1 -- Controlled Pressure Source (MA)/LConn2
  Heater/RConn2 -- PS Add/LConn1 -- CO2_1/RConn2 -- Bed Temp 1/RConn1
  Simulink-PS Converter2/RConn1 -- PS Gain1/LConn1
  Volumetric Flow Rate Sensor (MA) Upstream/RConn2 -- PS-Simulink Converter7/LConn1
  PS-Simulink Converter1/LConn1 -- Mass & Energy Flow Rate Sensor (MA)/LConn3
  Heater/LConn1 -- htr_signal/RConn1
  Sorbent Bed2/LConn1 -- Sorbent Bed1/RConn1
  Sorbent Bed/RConn1 -- Sorbent Bed1/LConn1
  Heater/RConn1 -- CO2_2/RConn2 -- PS Add/LConn2 -- Bed Temp 2/RConn1
  Heater/RConn3 -- CO2_3/RConn2 -- PS Add1/LConn2 -- Bed Temp 3/RConn1
  Heater/LConn4 -- Sorbent Bed1/LConn2 -- Conductive Heat Transfer5/LConn1 -- Conductive Heat Transfer7/LConn1 -- Conductive Heat Transfer4/LConn1 -- Conductive Heat Transfer8/LConn1
  Conductive Heat Transfer9/LConn1 -- Heater/RConn4 -- Sorbent Bed2/LConn2 -- Conductive Heat Transfer5/RConn1 -- Conductive Heat Transfer7/RConn1 -- Conductive Heat Transfer10/LConn1
  Measurement Selector (MA)2/RConn2 -- Bed out Temp/RConn1
  Pipe (MA)1/LConn1 -- Mass & Energy Flow Rate Sensor (MA)/RConn1
  Measurement Selector (MA)3/RConn2 -- "Bed in Temp "/RConn1 -- CO2 Adsorption/RConn1
  Pipe (MA)6/RConn1 -- Controlled Pressure Source (MA)/LConn1 -- Pressure & Temperature Sensor (MA)/LConn1
  Pipe (MA)6/LConn1 -- Sorbent Bed2/RConn1
  Pipe (MA)6/LConn2 -- Conductive Heat Transfer6/LConn1 -- Conductive Heat Transfer3/RConn1 -- Thermal Mass1/LConn1
  Measurement Selector (MA)3/LConn1 -- Pipe (MA)1/RConn3
  Measurement Selector (MA)2/LConn1 -- Pipe (MA)6/RConn3
  sig/RConn1 -- PS-Simulink Converter9/LConn1
  Measurement Selector (MA)3/RConn4 -- Bed in Mole fraction/RConn1 -- PS-Simulink Converter3/LConn1
  Pipe (MA)1/RConn1 -- Sorbent Bed/LConn1
  CO2 on/off/RConn1 -- PS Switch2/LConn3 -- PS Switch/LConn3 -- PS Switch1/LConn2 -- CO2 Adsorption/RConn3 -- CO2 Desorption/LConn2
  PS-Simulink Converter10/LConn1 -- Measurement Selector (MA)/RConn4
  PS Switch1/LConn3 -- PS Gain1/RConn1 -- Des CO2/RConn1
  PS Switch1/LConn1 -- CO2 Adsorption/RConn2
  PS Switch/LConn1 -- Des_sig/RConn1
  PS Constant/RConn1 -- PS Switch/LConn2
  PS Switch/RConn1 -- CO2 Desorption/LConn1
  PS Switch2/LConn1 -- Cycle_end_sig/RConn1
  PS Constant1/RConn1 -- PS Switch2/LConn2
  PS Switch2/RConn1 -- PS-Simulink Converter8/LConn1
  Convective Heat Transfer/LConn1 -- Radiative Heat Transfer1/LConn1 -- Conductive Heat Transfer1/RConn1
  Radiative Heat Transfer1/RConn1 -- Convective Heat Transfer/RConn1 -- Temperature Source1/LConn1
  Convective Heat Transfer1/RConn1 -- Radiative Heat Transfer/RConn1 -- Temperature Source6/LConn1
  Convective Heat Transfer1/LConn1 -- Radiative Heat Transfer/LConn1 -- Conductive Heat Transfer6/RConn1
  CO2_1/LConn1 -- Sorbent Bed/LConn3
  Thermal Reference7/LConn1 -- Temperature Sensor1/RConn1
  PS-Simulink Converter11/LConn1 -- Temperature Sensor1/RConn2
  CO2_2/LConn1 -- Sorbent Bed1/LConn3
  CO2_3/LConn1 -- Sorbent Bed2/LConn3
  PS Switch1/RConn1 -- Heater/LConn2 -- PS Divide/LConn1
  PS Divide/RConn1 -- CO2_1/RConn1 -- CO2_2/RConn1 -- CO2_3/RConn1
  PS Constant2/RConn1 -- PS Divide/LConn2
  PS Add1/LConn1 -- PS Add/RConn1
  PS Divide1/LConn1 -- PS Add1/RConn1
  PS Constant3/RConn1 -- PS Divide1/LConn2
  PS Divide1/RConn1 -- PS-Simulink Converter5/LConn1 -- CO2 Adsorption/LConn1
  Conductive Heat Transfer1/LConn1 -- Conductive Heat Transfer2/RConn1 -- Pipe (MA)1/LConn2 -- Thermal Mass2/LConn1 -- Temperature Sensor1/LConn1
  Conductive Heat Transfer9/RConn1 -- Conductive Heat Transfer10/RConn1 -- Conductive Heat Transfer3/LConn1
  Conductive Heat Transfer4/RConn1 -- Conductive Heat Transfer11/LConn1 -- Conductive Heat Transfer12/LConn1 -- Sorbent Bed/LConn2 -- Heater/LConn3 -- Conductive Heat Transfer8/RConn1
  Conductive Heat Transfer12/RConn1 -- Conductive Heat Transfer11/RConn1 -- Conductive Heat Transfer2/LConn1
